simulink model "model2"  (R2023b)
settings: Solver=VariableStepAuto  StartTime=0.0  StopTime=2500  RelTol=1e-3
values from neighbouring files (symbols this model uses):
  A = double(subs(A, [q0, g, h1, h2, p1, p2, s1, s2, R1, R2, S2, S1],      [q0_, g_, h1_, h2_, p1_, p2_, s1_, s2_, R1_, R2_, S2_, S1_]))    [new_lin.m]
  B = double(subs(B, [q0, g, h1, h2, p1, p2, s1, s2, R1, R2, S2, S1],      [q0_, g_, h1_, h2_, p1_, p2_, s1_, s2_, R1_, R2_, S2_, S1_]))    [new_lin.m]
  g_ = 9.81    [new_lin.m]
  h1_ = 0.15    [new_lin.m]
  h2_ = (a^2*h1_)/(b^2)    [new_lin.m]
  p1_ = 0.85    [new_lin.m]
  p2_ = 0.95    [new_lin.m]
  q0_ = b*sqrt(h2_)    [new_lin.m]
  s1_ = 0.083    [new_lin.m]
  S1_ = 2*pi*R1_*h1_ + 2*pi*R1_^2    (= 27.0176968209)    [new_lin.m]
  s2_ = 0.083    [new_lin.m]
  S2_ = 2*pi*R2_*h2_ + 2*pi*R2_^2    [new_lin.m]
settings Model: Creator=ralex  LastModifiedBy=ralex

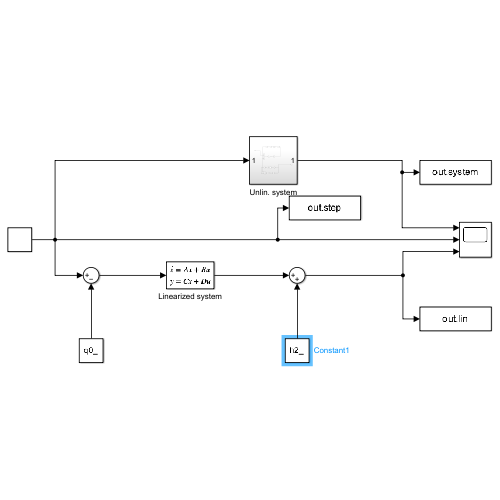
[thumbnail: Simulink's stored preview of the top-level diagram]
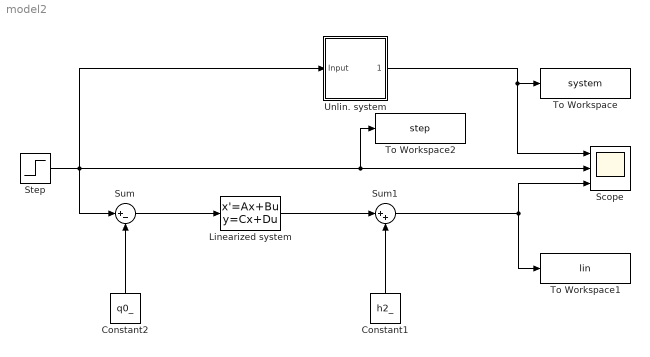
== system model2 ==
  Constant1 : Constant  Value=h2_
  Constant2 : Constant  Value=q0_
  Linearized system : StateSpace  A=A  B=B  C=[0 1]  D=0  InitialCondition=[0 0]
  Scope : Scope  NumInputPorts=3
  Step : Step  Time=200  Before=q0_  After=q0_*1.1  SampleTime=0
  Sum : Sum  Inputs=|+-
  Sum1 : Sum  Inputs=|++
  To Workspace : ToWorkspace  VariableName=system  SaveFormat=Timeseries  SampleTime=-1
  To Workspace1 : ToWorkspace  VariableName=lin  SaveFormat=Timeseries  SampleTime=-1
  To Workspace2 : ToWorkspace  VariableName=step  SaveFormat=Timeseries  SampleTime=-1
  Unlin. system : Subsystem
  wires:
  Sum1/1 -> To Workspace1/1, Scope/3
  Constant1/1 -> Sum1/2
  Step/1 -> Unlin. system/1(Input), Sum/1, To Workspace2/1, Scope/2
  Unlin. system/1(Output) -> Scope/1, To Workspace/1
  Linearized system/1 -> Sum1/1
  Sum/1 -> Linearized system/1
  Constant2/1 -> Sum/2

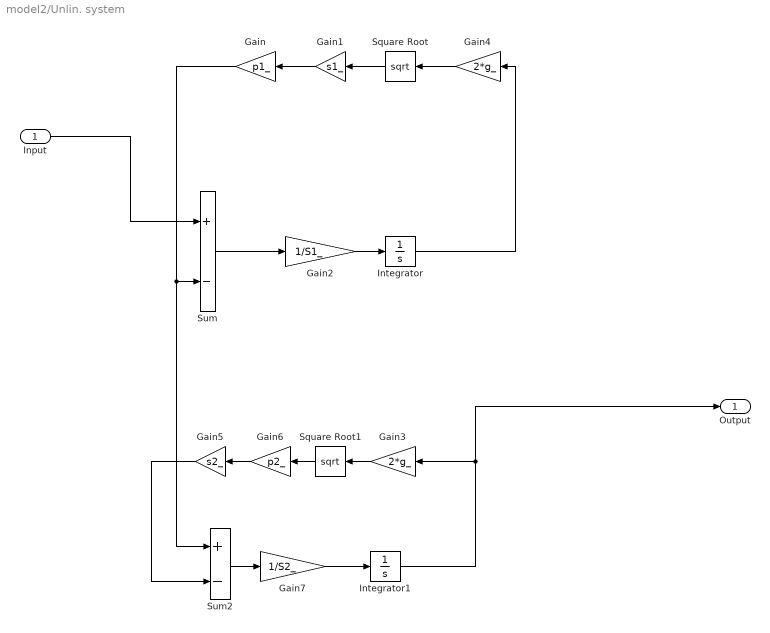
== system model2/Unlin. system ==
  Input : Inport
  Gain : Gain  Gain=p1_
  Gain1 : Gain  Gain=s1_
  Gain2 : Gain  Gain=1/S1_
  Gain3 : Gain  Gain=2*g_
  Gain4 : Gain  Gain=2*g_
  Gain5 : Gain  Gain=s2_
  Gain6 : Gain  Gain=p2_
  Gain7 : Gain  Gain=1/S2_
  Integrator : Integrator  InitialCondition=h1_
  Integrator1 : Integrator  InitialCondition=h2_
  Square Root : Sqrt
  Square Root1 : Sqrt
  Sum : Sum  Inputs=+-
  Sum2 : Sum  Inputs=+-
  Output : Outport
  wires:
  Gain/1 -> Sum/2, Sum2/1
  Gain1/1 -> Gain/1
  Input/1 -> Sum/1
  Integrator/1 -> Gain4/1
  Square Root/1 -> Gain1/1
  Gain4/1 -> Square Root/1
  Gain5/1 -> Sum2/2
  Sum/1 -> Gain2/1
  Integrator1/1 -> Output/1, Gain3/1
  Gain6/1 -> Gain5/1
  Square Root1/1 -> Gain6/1
  Gain3/1 -> Square Root1/1
  Sum2/1 -> Gain7/1
  Gain2/1 -> Integrator/1
  Gain7/1 -> Integrator1/1
